simulink model "firmware"  (R2020a)
settings: Solver=FixedStepAuto  StartTime=0.0  StopTime=10.0  FixedStep=1e-3  RelTol=1e-3  EnableMultiTasking=on
undefined symbols (not defined in the file): A0, A1, D0, D1, D10, D11, D12, D13, D2, D3, D4, D5, D6, D7, D8, D9, magnitude, PTA0, PTA1, PTA2, PTB2, PTB23, PTB3, PTB9, PTC16, PTC17, PTC2, PTC3, PTC4, PTD0, PTD1, PTD2, PTD3
libraries: etargetslib x35, frdmk64flib x23, dspstat3 x1
(part 2 of 2)

== stateflow chart firmware/Pacemaker Control ==
  state AOO
    state Shock
      entry:
      paceAtrium = true;
      exit:
      paceAtrium = false;
    state Prep
      entry:
      preparePaceAtrium = true;
      exit:
      preparePaceAtrium = false;
    (default) -> AOO.Prep
    AOO.Prep -> AOO.Shock : [after(maximumLimit-atrialPulseWidth,msec)]
    AOO.Shock -> AOO.Prep : [after(atrialPulseWidth,msec)]
  state VOO
    state Shock
      entry:
      paceVentricle = true;
      exit:
      paceVentricle = false;
    state Prep
      entry:
      preparePaceVentricle = true;
      exit:
      preparePaceVentricle = false;
    (default) -> VOO.Prep
    VOO.Prep -> VOO.Shock : [after(maximumLimit-ventricularPulseWidth,msec)]
    VOO.Shock -> VOO.Prep : [after(ventricularPulseWidth,msec)]
  state Off
    entry:
    reset = true;
    preparePaceAtrium = false;
    paceAtrium = false;
    preparePaceVentricle = false;
    paceVentricle = false;
    sense = false;
    exit:
    reset = false;
  state VOOR
    state Shock
      entry:
      paceVentricle = true;
      exit:
      paceVentricle = false;
    state Prep
      entry:
      preparePaceVentricle = true;
      exit:
      preparePaceVentricle = false;
    (default) -> VOOR.Prep
    VOOR.Prep -> VOOR.Shock : [after(rateAdaptiveLimit-ventricularPulseWidth,msec)]
    VOOR.Shock -> VOOR.Prep : [after(ventricularPulseWidth,msec)]
  state Initialize
    entry:
    AOO = 100;
    VOO = 200;
    AAI = 111;
    VVI = 221;
    AOOR = 109;
    VOOR = 209;
    AAIR = 120;
    VVIR = 230;
    DDD = 33;
    DDDR = 42;
  state AOOR
    state Shock
      entry:
      paceAtrium = true;
      exit:
      paceAtrium = false;
    state Prep
      entry:
      preparePaceAtrium = true;
      exit:
      preparePaceAtrium = false;
    (default) -> AOOR.Prep
    AOOR.Prep -> AOOR.Shock : [after(rateAdaptiveLimit-atrialPulseWidth,msec)]
    AOOR.Shock -> AOOR.Prep : [after(atrialPulseWidth,msec)]
  state DDD
    state ShockAtrium
      entry:
      t = 0;
      paceAtrium = true;
      sense = true;
      during:
      t = t+1;
      exit:
      paceAtrium = false;
    state PrepAtrium
      entry:
      preparePaceAtrium = true;
      sense = true;
      exit:
      preparePaceAtrium = false;
    state ShockAtrium_SensedVentricle
      entry:
      paceAtrium = true;
      during:
      exit:
      t = 0;
      paceAtrium = false;
    state Reset3
      entry:
      reset = true;
      exit:
      reset = false;
    state Reset2
      entry:
      reset = true;
      exit:
      reset = false;
    state SensedAtrium
      entry:
      preparePaceVentricle = true;
      exit:
      preparePaceVentricle = false;
    state DischargeBlockingCapA
      entry:
      t = 0;
      preparePaceAtrium = true;
      sense = true;
      during:
      t = t+1;
      exit:
      preparePaceAtrium = false;
    state DischargeBlockingCapA_SensedVentricle
      entry:
      preparePaceAtrium = true;
      during:
      exit:
      t = 0;
      preparePaceAtrium = false;
    state DischargeBlockingCapV
      entry:
      preparePaceVentricle = true;
      exit:
      preparePaceVentricle = false;
    state Reset1
      entry:
      reset = true;
      exit:
      reset = false;
    state PrepVentricle
      entry:
      t = 0;
      preparePaceVentricle = true;
      sense = true;
      during:
      t = t+1;
      exit:
      preparePaceVentricle = false;
    state ShockVentricle
      entry:
      paceVentricle = true;
      exit:
      paceVentricle = false;
    (default) -> DDD.PrepAtrium
    DDD.PrepAtrium -> DDD.ShockAtrium [order 1] : [after(maximumLimit-(3*AVDelay+ventricularPulseWidth)/2,msec)]
    DDD.ShockAtrium -> DDD.ShockAtrium_SensedVentricle [order 2] : [ventricularSignalDetected || button]
    DDD.PrepAtrium -> DDD.Reset3 [order 2] : [atrialSignalDetected]
    DDD.Reset2 -> DDD.PrepAtrium
    DDD.ShockAtrium -> DDD.DischargeBlockingCapA [order 1] : [after(atrialPulseWidth,msec)]
    DDD.Reset3 -> DDD.SensedAtrium
    DDD.ShockAtrium_SensedVentricle -> DDD.DischargeBlockingCapA_SensedVentricle : [after(atrialPulseWidth-t,msec)]
    DDD.SensedAtrium -> DDD.Reset2 [order 2] : [ventricularSignalDetected || button]
    DDD.DischargeBlockingCapV -> DDD.Reset2 : [after((AVDelay-ventricularPulseWidth)/2,msec)]
    (junction 208) -> DDD.Reset2 : [after(AVDelay+(ventricularPulseWidth - atrialPulseWidth)/2 - t, msec)]
    DDD.DischargeBlockingCapA -> DDD.DischargeBlockingCapA_SensedVentricle [order 2] : [ventricularSignalDetected || button]
    DDD.SensedAtrium -> DDD.ShockVentricle [order 1] : [after(AVDelay,msec)]
    DDD.DischargeBlockingCapA_SensedVentricle -> (junction 208) : [after((AVDelay-atrialPulseWidth)/2-t, msec)]
    DDD.DischargeBlockingCapA -> DDD.Reset1 [order 1] : [after((AVDelay-atrialPulseWidth)/2, msec)]
    DDD.ShockVentricle -> DDD.DischargeBlockingCapV : [after(ventricularPulseWidth, msec)]
    DDD.Reset1 -> DDD.PrepVentricle
    DDD.PrepVentricle -> (junction 208) [order 2] : [ventricularSignalDetected || button]
    DDD.PrepVentricle -> DDD.ShockVentricle [order 1] : [after((AVDelay-atrialPulseWidth)/2, msec)]
  state DDDR
    state ShockAtrium
      entry:
      t = 0;
      paceAtrium = true;
      sense = true;
      during:
      t = t+1;
      exit:
      paceAtrium = false;
    state PrepAtrium
      entry:
      preparePaceAtrium = true;
      sense = true;
      exit:
      preparePaceAtrium = false;
    state ShockAtrium_SensedVentricle
      entry:
      paceAtrium = true;
      during:
      exit:
      t = 0;
      paceAtrium = false;
    state Reset3
      entry:
      reset = true;
      exit:
      reset = false;
    state Reset2
      entry:
      reset = true;
      exit:
      reset = false;
    state SensedAtrium
      entry:
      preparePaceVentricle = true;
      exit:
      preparePaceVentricle = false;
    state DischargeBlockingCapA
      entry:
      t = 0;
      preparePaceAtrium = true;
      sense = true;
      during:
      t = t+1;
      exit:
      preparePaceAtrium = false;
    state DischargeBlockingCapA_SensedVentricle
      entry:
      preparePaceAtrium = true;
      during:
      exit:
      t = 0;
      preparePaceAtrium = false;
    state DischargeBlockingCapV
      entry:
      preparePaceVentricle = true;
      exit:
      preparePaceVentricle = false;
    state Reset1
      entry:
      reset = true;
      exit:
      reset = false;
    state PrepVentricle
      entry:
      t = 0;
      preparePaceVentricle = true;
      sense = true;
      during:
      t = t+1;
      exit:
      preparePaceVentricle = false;
    state ShockVentricle
      entry:
      paceVentricle = true;
      exit:
      paceVentricle = false;
    (default) -> DDDR.PrepAtrium
    DDDR.PrepAtrium -> DDDR.ShockAtrium [order 1] : [after(rateAdaptiveLimit-(3*AVDelay+ventricularPulseWidth)/2,msec)]
    DDDR.ShockAtrium -> DDDR.ShockAtrium_SensedVentricle [order 2] : [ventricularSignalDetected || button]
    DDDR.PrepAtrium -> DDDR.Reset3 [order 2] : [atrialSignalDetected]
    DDDR.Reset2 -> DDDR.PrepAtrium
    DDDR.ShockAtrium -> DDDR.DischargeBlockingCapA [order 1] : [after(atrialPulseWidth,msec)]
    DDDR.Reset3 -> DDDR.SensedAtrium
    DDDR.ShockAtrium_SensedVentricle -> DDDR.DischargeBlockingCapA_SensedVentricle : [after(atrialPulseWidth-t,msec)]
    DDDR.SensedAtrium -> DDDR.Reset2 [order 2] : [ventricularSignalDetected || button]
    DDDR.DischargeBlockingCapV -> DDDR.Reset2 : [after((AVDelay-ventricularPulseWidth)/2,msec)]
    (junction 226) -> DDDR.Reset2 : [after(AVDelay+(ventricularPulseWidth - atrialPulseWidth)/2 - t, msec)]
    DDDR.DischargeBlockingCapA -> DDDR.DischargeBlockingCapA_SensedVentricle [order 2] : [ventricularSignalDetected || button]
    DDDR.SensedAtrium -> DDDR.ShockVentricle [order 1] : [after(AVDelay,msec)]
    DDDR.DischargeBlockingCapA_SensedVentricle -> (junction 226) : [after((AVDelay-atrialPulseWidth)/2-t, msec)]
    DDDR.DischargeBlockingCapA -> DDDR.Reset1 [order 1] : [after((AVDelay-atrialPulseWidth)/2, msec)]
    DDDR.ShockVentricle -> DDDR.DischargeBlockingCapV : [after(ventricularPulseWidth, msec)]
    DDDR.Reset1 -> DDDR.PrepVentricle
    DDDR.PrepVentricle -> (junction 226) [order 2] : [ventricularSignalDetected || button]
    DDDR.PrepVentricle -> DDDR.ShockVentricle [order 1] : [after((AVDelay-atrialPulseWidth)/2, msec)]
  state AAIR
    state SenseDelay
      entry:
      preparePaceAtrium = true;
      sense = true;
      exit:
      preparePaceAtrium = false;
    state Pace
      entry:
      paceAtrium = true;
      exit:
      paceAtrium = false;
    state SenseNoDelay
      entry:
      preparePaceAtrium = true;
      sense = true;
      exit:
      preparePaceAtrium = false;
    AAIR.SenseDelay -> AAIR.SenseDelay [order 2] : [atrialSignalDetected && after(100,msec)]
    AAIR.SenseDelay -> AAIR.Pace [order 1] : [after(rateAdaptiveLimit, msec) && after(ARP, msec)]
    AAIR.SenseNoDelay -> AAIR.SenseDelay [order 1] : [atrialSignalDetected]
    AAIR.SenseNoDelay -> AAIR.Pace [order 2] : [after(rateAdaptiveLimit, msec) && after(ARP, msec)]
    (default) -> AAIR.SenseNoDelay
    AAIR.Pace -> AAIR.SenseNoDelay : [after(atrialPulseWidth,msec)]
  state VVIR
    state SenseDelay
      entry:
      preparePaceVentricle = true;
      sense = true;
      exit:
      preparePaceVentricle = false;
    state Pace
      entry:
      paceVentricle = true;
      exit:
      paceVentricle = false;
    state Sense
      entry:
      preparePaceVentricle = true;
      sense = true;
      exit:
      preparePaceVentricle = false;
    VVIR.SenseDelay -> VVIR.SenseDelay [order 1] : [ventricularSignalDetected && after(100,msec)]
    VVIR.SenseDelay -> VVIR.Pace [order 2] : [after(rateAdaptiveLimit, msec) && after(VRP, msec)]
    VVIR.Sense -> VVIR.SenseDelay [order 2] : [ventricularSignalDetected]
    VVIR.Sense -> VVIR.Pace [order 1] : [after(rateAdaptiveLimit, msec) && after(VRP, msec)]
    (default) -> VVIR.Sense
    VVIR.Pace -> VVIR.Sense : [after(ventricularPulseWidth, msec)]
  state AAI
    state SenseDelay
      entry:
      preparePaceAtrium = true;
      sense = true;
      exit:
      preparePaceAtrium = false;
    state Pace
      entry:
      paceAtrium = true;
      exit:
      paceAtrium = false;
    state SenseNoDelay
      entry:
      preparePaceAtrium = true;
      sense = true;
      exit:
      preparePaceAtrium = false;
    AAI.SenseDelay -> AAI.SenseDelay [order 2] : [atrialSignalDetected && after(100,msec)]
    AAI.SenseDelay -> AAI.Pace [order 1] : [after(maximumLimit, msec) && after(ARP, msec)]
    AAI.SenseNoDelay -> AAI.SenseDelay [order 1] : [atrialSignalDetected]
    AAI.SenseNoDelay -> AAI.Pace [order 2] : [after(maximumLimit, msec) && after(ARP, msec)]
    (default) -> AAI.SenseNoDelay
    AAI.Pace -> AAI.SenseNoDelay : [after(atrialPulseWidth,msec)]
  state VVI
    state SenseDelay
      entry:
      preparePaceVentricle = true;
      sense = true;
      exit:
      preparePaceVentricle = false;
    state Pace
      entry:
      paceVentricle = true;
      exit:
      paceVentricle = false;
    state Sense
      entry:
      preparePaceVentricle = true;
      sense = true;
      exit:
      preparePaceVentricle = false;
    VVI.SenseDelay -> VVI.SenseDelay [order 1] : [ventricularSignalDetected && after(100,msec)]
    VVI.SenseDelay -> VVI.Pace [order 2] : [after(maximumLimit, msec) && after(VRP, msec)]
    VVI.Sense -> VVI.SenseDelay [order 2] : [ventricularSignalDetected]
    VVI.Sense -> VVI.Pace [order 1] : [after(maximumLimit, msec) && after(VRP, msec)]
    (default) -> VVI.Sense
    VVI.Pace -> VVI.Sense : [after(ventricularPulseWidth, msec)]
  AOO -> Off : [mode ~= AOO]
  Off -> AOO [order 3] : [mode ==AOO]
  Off -> VOO [order 4] : [mode == VOO]
  VOO -> Off : [mode ~= VOO]
  Off -> VOOR [order 6] : [mode == VOOR]
  Off -> AOOR [order 5] : [mode == AOOR]
  VOOR -> Off : [mode ~= VOOR]
  AOOR -> Off : [mode ~= AOOR]
  (default) -> Initialize
  Off -> DDD [order 9] : [mode == DDD]
  DDD -> Off : [mode ~= DDD]
  Initialize -> Off
  DDDR -> Off : [mode ~= DDDR]
  Off -> DDDR [order 10] : [mode == DDDR]
  AAIR -> Off : [mode ~= AAIR]
  VVIR -> Off : [mode~=VVIR]
  Off -> AAIR [order 7] : [mode == AAIR]
  Off -> VVIR [order 8] : [mode == VVIR]
  AAI -> Off : [mode ~= AAI]
  Off -> AAI [order 1] : [mode == AAI]
  VVI -> Off : [mode ~= VVI]
  Off -> VVI [order 2] : [mode == VVI]
  data: preparePaceAtrium output; paceAtrium output; preparePaceVentricle output; paceVentricle output; mode input; reset output; atrialSignalDetected input; ventricularSignalDetected input; maximumLimit input; atrialPulseWidth input; ventricularPulseWidth input; VRP input; ARP input; sense output; AAI local; AOO local; AAIR local; AOOR local; DDD local; DDDR local; VOO local; VOOR local; VVI local; VVIR local; rateAdaptiveLimit input; AVDelay input; t local; button input

== stateflow chart firmware/Outputs/LED Pin Control ==
  state Initialize
    entry:
    Off = 0;
    AOO = 100;
    VOO = 200;
    AAI = 111;
    VVI = 221;
    AOOR = 109;
    VOOR = 209;
    AAIR = 120;
    VVIR = 230;
    DDD = 33;
    DDDR = 42;
    delay = 1;
  state DDD
    entry:
    r = false;
    g = true;
    b = true;
  state DDDR
    entry:
    r = false;
    g = false;
    b = false;
  state Off
    entry:
    r = true;
    g = true;
    b = true;
  state AOOR
    entry:
    r = false;
    g = false;
    b = false;
  state AOO
    entry:
    r = true;
    g = false;
    b = false;
  state VVI
    entry:
    r = false;
    g = false;
    b = true;
  state VVIR
    entry:
    r = false;
    g = false;
    b = false;
  state AAI
    entry:
    r = true;
    g = false;
    b = true;
  state AAIR
    entry:
    r = false;
    g = false;
    b = false;
  state VOOR
    entry:
    r = false;
    g = false;
    b = false;
  state VOO
    entry:
    r = false;
    g = true;
    b = false;
  (default) -> Initialize
  DDD -> DDDR [order 2] : [mode == DDDR && after(delay,sec)]
  Initialize -> Off
  DDD -> Off [order 1] : [mode ~= DDD && mode ~= DDDR]
  DDDR -> DDD : [after(delay,sec)]
  Off -> AOO : [mode ~= Off]
  VVI -> DDD [order 1] : [mode ~= VVI && mode ~= VVIR]
  AOO -> AOOR [order 2] : [mode == AOOR && after(delay, sec)]
  VVI -> VVIR [order 2] : [mode == VVIR && after(delay,sec)]
  AOOR -> AOO : [after(delay, sec)]
  VVIR -> VVI : [after(delay,sec)]
  AAI -> VVI [order 1] : [mode ~= AAI && mode ~= AAIR]
  AOO -> VOO [order 1] : [mode ~= AOO && mode ~= AOOR]
  AAI -> AAIR [order 2] : [mode == AAIR && after(delay,sec)]
  VOO -> VOOR [order 2] : [mode == VOOR && after(delay,sec)]
  VOO -> AAI [order 1] : [mode ~= VOO && mode ~= VOOR]
  VOOR -> VOO : [after(delay,sec)]
  AAIR -> AAI : [after(delay,sec)]
  data: mode input; r output; g output; b output; AAIR local; AOOR local; DDD local; DDDR local; VOOR local; VVIR local; AAI local; AOO local; Off local; VOO local; VVI local; delay local

== stateflow chart firmware/Outputs/Sensing Pin Control ==
  state Sense
    entry:
    VENT_CMP_REF_PWM = ventricularSensitivityDutyCycle;
    ATR_CMP_REF_PWM = atrialSensitivityDutyCycle;
    FRONT_END_CTRL = true;
  state Default
    entry:
    %Set all pins to 0/false
    FRONT_END_CTRL = true;
    VENT_CMP_REF_PWM = 0;
    ATR_CMP_REF_PWM = 0;
  Default -> Sense : [sense]
  Sense -> Default : [~sense]
  (default) -> Default
  data: FRONT_END_CTRL output; sense input; atrialSensitivityDutyCycle input; ventricularSensitivityDutyCycle input; ATR_CMP_REF_PWM output; VENT_CMP_REF_PWM output

== stateflow chart firmware/Serial Communication/EGRAM CLOCK ==
  state Send_EGRAM
    entry:
    send_message(5);
  state Waiting
  (default) -> Waiting
  Waiting -> Send_EGRAM : [msg_ready && egram_status ~= 0]
  Send_EGRAM -> Waiting
  data: egram_status input; msg_ready input

== stateflow chart firmware/Serial Communication/EGRAM DATA COLLECTOR ==
  state Start
    wait = 2;
  state TimeStep1
    entry:
    as1 = atrialAnalogSignal;
    vs1 = ventricularAnalogSignal;
    msg_ready = false;
  state TimeStep2
    entry:
    as2 = atrialAnalogSignal;
    vs2 = ventricularAnalogSignal;
    msg_ready = false;
  state TimeStep3
    entry:
    as3 = atrialAnalogSignal;
    vs3 = ventricularAnalogSignal;
    msg_ready = false;
  state TimeStep4
    entry:
    as4 = atrialAnalogSignal;
    vs4 = ventricularAnalogSignal;
    msg_ready = false;
  state TimeStep5
    entry:
    as5 = atrialAnalogSignal;
    vs5 = ventricularAnalogSignal;
    msg_ready = false;
  state TimeStep6
    entry:
    as6 = atrialAnalogSignal;
    vs6 = ventricularAnalogSignal;
    msg_ready = false;
  state Send
    entry:
    as10 = atrialAnalogSignal;
    vs10 = ventricularAnalogSignal;
    msg_ready = true;
  state TimeStep7
    entry:
    as7 = atrialAnalogSignal;
    vs7 = ventricularAnalogSignal;
    msg_ready = false;
  state TimeStep9
    entry:
    as9 = atrialAnalogSignal;
    vs9 = ventricularAnalogSignal;
    msg_ready = false;
  state TimeStep8
    entry:
    as8 = atrialAnalogSignal;
    vs8 = ventricularAnalogSignal;
    msg_ready = false;
  (default) -> Start
  Start -> TimeStep1
  TimeStep2 -> TimeStep3 : [after(wait,msec)]
  TimeStep3 -> TimeStep4 : [after(wait,msec)]
  TimeStep4 -> TimeStep5 : [after(wait,msec)]
  TimeStep1 -> TimeStep2 : [after(wait,msec)]
  TimeStep5 -> TimeStep6 : [after(wait,msec)]
  Send -> TimeStep1 : [after(wait,msec)]
  TimeStep6 -> TimeStep7 : [after(wait,msec)]
  TimeStep9 -> Send : [after(wait,msec)]
  TimeStep7 -> TimeStep8 : [after(wait,msec)]
  TimeStep8 -> TimeStep9 : [after(wait,msec)]
  data: atrialAnalogSignal input; ventricularAnalogSignal input; msg_ready output; as1 output; as2 output; as3 output; vs1 output; vs2 output; vs3 output; as10 output; as4 output; as5 output; as6 output; as7 output; as8 output; as9 output; vs10 output; vs4 output; vs5 output; vs6 output; vs7 output; vs8 output; vs9 output; wait local

== stateflow chart firmware/Inputs/Rate Adaptive Subsystem/Accel to Activity/Chart ==
  state start
    entry:
    activity = 0;
  state pushActivity
    entry:
    activity = magnitude;
  state Wait
  (default) -> start
  start -> Wait
  pushActivity -> Wait
  Wait -> pushActivity : [after(1000,msec)]
  data: magnitude input; activity output

== stateflow chart firmware/Inputs/Rate Adaptive Subsystem/Decide HR ==
  state start
    entry:
    HR = LRL;
  state Increase
    entry:
    min = HR;
    max = MSR;
    t = 0;
    logScaling =  log(1 + scaling* Reaction_Time);
    during:
    t = t + increment;
    HR= min + (max - min)*((log(1 + scaling*t)) / logScaling);
  state Default
    entry:
    tolerance = 1
    scaling = 1;
    increment = 0.001;
  state Decreasing
    entry:
    scaling = 0.25;
    t = 0;
    max = HR;
    min = LRL;
    during:
    logScaling = log(1+scaling*Recovery_Time);
    t = t + increment;
    HR= max - (max - min)*((log(1 + scaling*t)) / logScaling);
  state AtMax
    entry:
    HR = MSR;
  state AtMin
    entry:
    HR = LRL;
  state ActiveDecreasing
    entry:
    t = 0;
    logScaling = log(1+scaling*Recovery_Time);
    oldMSR = MSR;
    min = LRL;
    max = HR;
    during:
    t = t + increment;
    HR= max - (max - min)*((log(1 + scaling*t)) / logScaling);
  (default) -> start
  start -> Default
  Default -> Decreasing [order 2] : [~active]
  Increase -> Increase [order 3] : [MSR > max]
  Default -> Increase [order 1] : [active]
  Increase -> ActiveDecreasing [order 4] : [HR > MSR]
  Decreasing -> Default [order 1] : [active]
  Increase -> Default [order 1] : [~active]
  ActiveDecreasing -> Increase [order 4] : [HR < MSR]
  (junction 16) -> Default
  Increase -> AtMax [order 2] : [HR >= MSR - tolerance]
  AtMax -> Increase [order 2] : [HR < MSR]
  Decreasing -> AtMin [order 2] : [HR <= LRL + tolerance]
  AtMax -> (junction 16) [order 1] : [~active]
  AtMin -> (junction 16) : [active]
  ActiveDecreasing -> (junction 16) [order 1] : [~active]
  ActiveDecreasing -> ActiveDecreasing [order 3] : [oldMSR > MSR && after(100,msec)]
  ActiveDecreasing -> AtMax [order 2] : [HR >= MSR - tolerance]
  AtMax -> ActiveDecreasing [order 3] : [HR > MSR]
  data: Recovery_Time input; Reaction_Time input; active input; MSR input; t local; tolerance local; LRL input; oldMSR local; logScaling local; min local; max local; scaling local; HR output; increment local

== stateflow chart firmware/Inputs/Rate Adaptive Subsystem/Is Active ==
  state isActive
    entry:
    isActive = true;
  state isNotActive
    entry:
    isActive = false;
  (default) -> isNotActive
  isActive -> isNotActive : [activity < Activity_Threshold]
  isNotActive -> isActive : [activity >= Activity_Threshold]
  data: Activity_Threshold input; activity input; isActive output
